simulink model "dyn"  (R2022a)
settings: Solver=VariableStepAuto  StartTime=0.0  StopTime=1.5  MaxStep=0.005  RelTol=1e-3
values from neighbouring files (symbols this model uses):
  A_1 = 0.0012    [WS.m]
  A_2 = 0.0012    [WS.m]
  D = [D_1 D_2 D_3 D_4 D_5 D_6]    [WS.m]
  E_1 = 8.25 * 10^4    (= 82500)    [WS.m]
  E_2 = 8.25 * 10^4    (= 82500)    [WS.m]
  g_x = 0.0    (= 0)    [WS.m]
  g_y = 0    [WS.m]
  g_z = 9.8    [WS.m]
  Gs_1 = E_1 / ( 2 * ( 1 + ni) )    (= 27684.5637584)    [WS.m]
  Gs_2 = E_2 / ( 2 *( 1 + ni) )    (= 27684.5637584)    [WS.m]
  Iax_1 = 1.0053e-07 * rate2    (= 9.55035e-08)    [WS.m]
  Iax_2 = 1.0053e-07 * rate2    (= 9.55035e-08)    [WS.m]
  Iay_1 = 1.0053e-07 * rate2    (= 9.55035e-08)    [WS.m]
  Iay_2 = 1.0053e-07 * rate2    (= 9.55035e-08)    [WS.m]
  Iaz_1 = 1.0053e-07 * rate2    (= 9.55035e-08)    [WS.m]
  Iaz_2 = 1.0053e-07 * rate2    (= 9.55035e-08)    [WS.m]
  Imx_1 = 10^-5 * rate1    (= 1e-05)    [WS.m]
  Imx_2 = 10^-5 * rate1    (= 1e-05)    [WS.m]
  Imy_1 = 10^-5 * rate1    (= 1e-05)    [WS.m]
  Imy_2 = 10^-5 * rate1    (= 1e-05)    [WS.m]
  Imz_1 = 10^-5 * rate1    (= 1e-05)    [WS.m]
  Imz_2 = 10^-5 * rate1    (= 1e-05)    [WS.m]
  l_1 = 0.05    [WS.m]
  l_2 = 0.05    [WS.m]
  m_1 = 0.08    [WS.m]
  m_2 = 0.08    [WS.m]
  p_tendon1_0 = [0.012,0,0]    [WS.m]
  p_tendon1_1 = [0.012,0,0]    [WS.m]
  p_tendon1_2 = [0.012,0,0]    [WS.m]
  p_tendon2_0 = [-0.012,0,0]    [WS.m]
  p_tendon2_1 = [-0.012,0,0]    [WS.m]
  p_tendon2_2 = [-0.012,0,0]    [WS.m]
  p_tendon3_0 = [0,0.012,0]    [WS.m]
  p_tendon3_1 = [0,0.012,0]    [WS.m]
  p_tendon3_2 = [0,0.012,0]    [WS.m]
  p_tendon4_0 = [0,-0.012,0]    [WS.m]
  p_tendon4_1 = [0,-0.012,0]    [WS.m]
  p_tendon4_2 = [0,-0.012,0]    [WS.m]
  p_tendon5_0 = [0.09,0,0]    [WS.m]
  p_tendon5_1 = [0.0636,0.0636,0]    [WS.m]
  p_tendon5_2 = [0,0.09,0]    [WS.m]
  x_0 = [0.001, 0.001 , 0.0 , 0 , 0.001,0]'    [WS.m]
  x_dot_0 = [0 , 0, 0, 0, 0, 0]'    [WS.m]
libraries: slpidlib x1, matrix_library x1
settings Model: Creator=atled  LastModifiedBy=atled

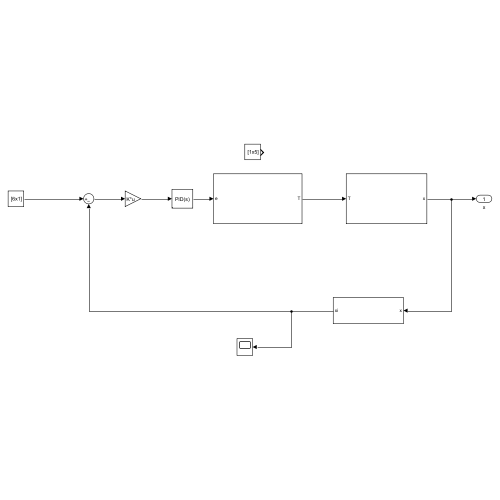
[thumbnail: Simulink's stored preview of the top-level diagram]
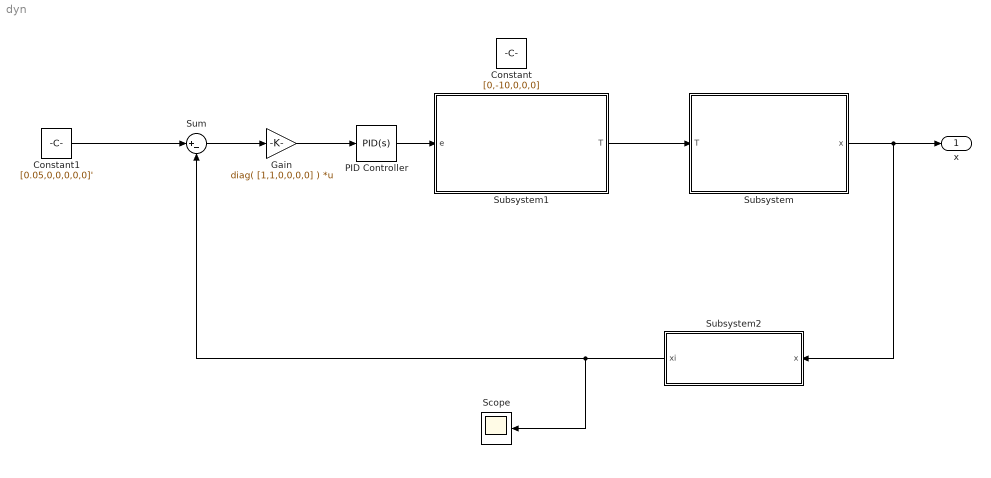
== system dyn ==
  Constant : Constant  Value=[0,-10,0,0,0]
  Constant1 : Constant  Value=[0.05,0,0,0,0,0]'  VectorParams1D=off
  Gain : Gain  Gain=diag( [1,1,0,0,0,0] )  Multiplication=Matrix(K*u)
  PID Controller : slpidlib/PID Controller  Controller=PID  Form=Parallel  TimeDomain=Continuous-time  UseExternalTs=off  SampleTime=-1  IntegratorMethod=Forward Euler  FilterMethod=Forward Euler  ControllerParametersSource=internal  P=0.2  I=0  UseKiTs=off  D=0  N=100  UseFilter=on  TunerSelectOption=Transfer Function Based (PID Tuner App)  InitialConditionSource=internal  InitialConditionForIntegrator=0  InitialConditionForFilter=0  DifferentiatorICPrevScaledInput=0  ExternalReset=none  TrackingMode=off  Kt=1  LimitOutput=off  SatLimitsSource=internal  UpperSaturationLimit=inf  LowerSaturationLimit=-inf  LinearizeAsGain=on  AntiWindupMode=none  Kb=1  POutMin=[]  POutMax=[]  IOutMin=[]  IOutMax=[]  DOutMin=[]  DOutMax=[]  NOutMin=[]  NOutMax=[]  SumOutMin=[]  SumOutMax=[]  SaturationOutMin=[]  SaturationOutMax=[]  PParamMin=[]  PParamMax=[]  IParamMin=[]  IParamMax=[]  DParamMin=[]  DParamMax=[]  NParamMin=[]  NParamMax=[]  KbParamMin=[]  KbParamMax=[]  KtParamMin=[]  KtParamMax=[]  KbOutMin=[]  KbOutMax=[]  KtOutMin=[]  KtOutMax=[]  IntegratorOutMin=[]  IntegratorOutMax=[]  FilterOutMin=[]  FilterOutMax=[]  SumI1OutMin=[]  SumI1OutMax=[]  SumI2OutMin=[]  SumI2OutMax=[]  SumI3OutMin=[]  SumI3OutMax=[]  SumI4OutMin=[]  SumI4OutMax=[]  SumDOutMin=[]  SumDOutMax=[]  DifferentiatorOutMin=[]  DifferentiatorOutMax=[]  FilterDiffOutCoefMin=[]  FilterDiffOutCoefMax=[]  ReciprocalOutMin=[]  ReciprocalOutMax=[]  SumDenOutMin=[]  SumDenOutMax=[]  SumNumOutMin=[]  SumNumOutMax=[]  DivideOutMin=[]  DivideOutMax=[]  UdiffTsProdOutMin=[]  UdiffTsProdOutMax=[]  NTsProdOutMin=[]  NTsProdOutMax=[]  UintegralTsProdOutMin=[]  UintegralTsProdOutMax=[]  UngainTsProdOutMin=[]  UngainTsProdOutMax=[]  IntegratorContinuousStateAttributes=''  IntegratorStateMustResolveToSignalObject=off  IntegratorRTWStateStorageClass=Auto  FilterContinuousStateAttributes=''  FilterStateMustResolveToSignalObject=off  FilterRTWStateStorageClass=Auto  ParallelPVariant=InternalParameters  IdealPVariant=Disabled  IVariant=InternalParameters  DVariant=InternalParameters  IntegratorVariant=Continuous  SatVariant=Disabled  AWVariant=Passthrough  PCopyVariant=Disabled  TRVariant=Disabled  FdbkBlocksVariant=Forward  IdealPFdbkVariant=Disabled  SatFdbkVariant=Disabled  DerivativeFilterVariant=ContFilter  NVariant=InternalParameters  NCopyVariant=Disabled  FilterICVariant=InternalICsFilter  IntegratorICVariant=InternalICs  ExternalResetVariant=Disabled  TRSumVariant=Passthrough  SumFdbkVariant=Disabled  SumVariant=Sum_PID  TsampFilterVariant=InternalTs  TsampNgainVariant=Passthrough  TsampIntegralVariant=Passthrough  ExternalSaturationOutDataTypeStr=Inherit: Same as second input  aMode=0
  Scope : Scope
  Subsystem : Subsystem
  Subsystem1 : Subsystem
  Subsystem2 : Subsystem
  Sum : Sum  Inputs=|+-
  x : Outport
  wires:
  Subsystem/1(x) -> Subsystem2/1(x), x/1
  Subsystem1/1(T) -> Subsystem/1(T)
  Constant1/1 -> Sum/1
  Subsystem2/1(xi) -> Sum/2, Scope/1
  Sum/1 -> Gain/1
  Gain/1 -> PID Controller/1
  PID Controller/1 -> Subsystem1/1(e)

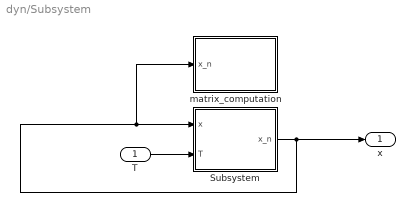
== system dyn/Subsystem ==
  T : Inport
  Subsystem : Subsystem
  matrix_computation : Subsystem
  x : Outport
  wires:
  Subsystem/1(x_n) -> x/1, matrix_computation/1(x_n), Subsystem/1(x)
  T/1 -> Subsystem/2(T)

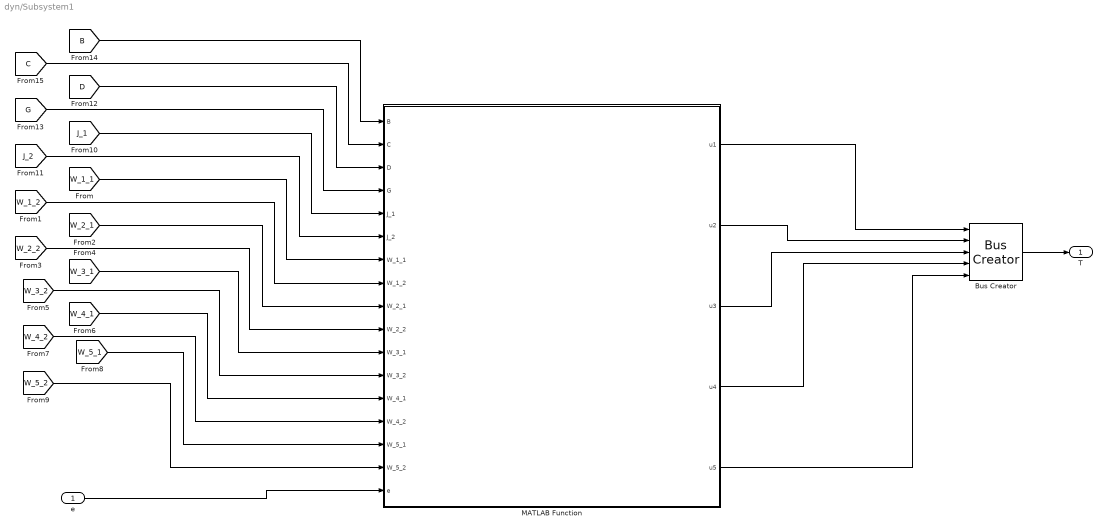
== system dyn/Subsystem1 ==
  e : Inport
  Bus Creator : BusCreator  Inputs=5
  MATLAB Function : MATLAB Function  TreatAsAtomicUnit=on
  T : Outport
  wires:
  [W_5_2] -> MATLAB Function/16(W_5_2)
  [W_4_1] -> MATLAB Function/13(W_4_1)
  [W_4_2] -> MATLAB Function/14(W_4_2)
  [J_2] -> MATLAB Function/6(J_2)
  [W_1_1] -> MATLAB Function/7(W_1_1)
  [G] -> MATLAB Function/4(G)
  [B] -> MATLAB Function/1(B)
  [J_1] -> MATLAB Function/5(J_1)
  [C] -> MATLAB Function/2(C)
  [D] -> MATLAB Function/3(D)
  [W_3_2] -> MATLAB Function/12(W_3_2)
  [W_2_2] -> MATLAB Function/10(W_2_2)
  e/1 -> MATLAB Function/17(e)
  [W_2_1] -> MATLAB Function/9(W_2_1)
  [W_3_1] -> MATLAB Function/11(W_3_1)
  [W_5_1] -> MATLAB Function/15(W_5_1)
  [W_1_2] -> MATLAB Function/8(W_1_2)
  MATLAB Function/1(u1) -> Bus Creator/1
  MATLAB Function/2(u2) -> Bus Creator/2
  MATLAB Function/3(u3) -> Bus Creator/3
  MATLAB Function/4(u4) -> Bus Creator/4
  MATLAB Function/5(u5) -> Bus Creator/5
  Bus Creator/1 -> T/1

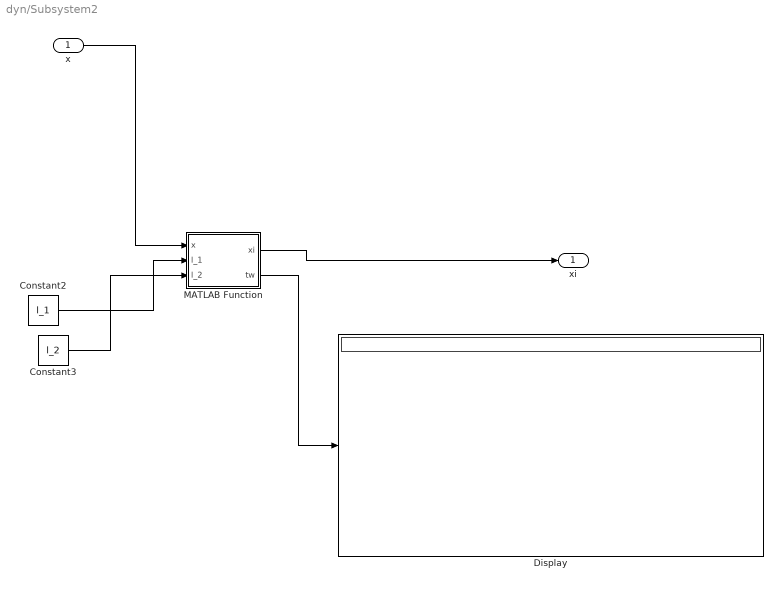
== system dyn/Subsystem2 ==
  x : Inport
  Constant2 : Constant  Value=l_1
  Constant3 : Constant  Value=l_2
  Display : Display
  MATLAB Function : MATLAB Function  TreatAsAtomicUnit=on
  xi : Outport
  wires:
  x/1 -> MATLAB Function/1(x)
  Constant3/1 -> MATLAB Function/3(l_2)
  MATLAB Function/1(xi) -> xi/1
  Constant2/1 -> MATLAB Function/2(l_1)
  MATLAB Function/2(tw) -> Display/1

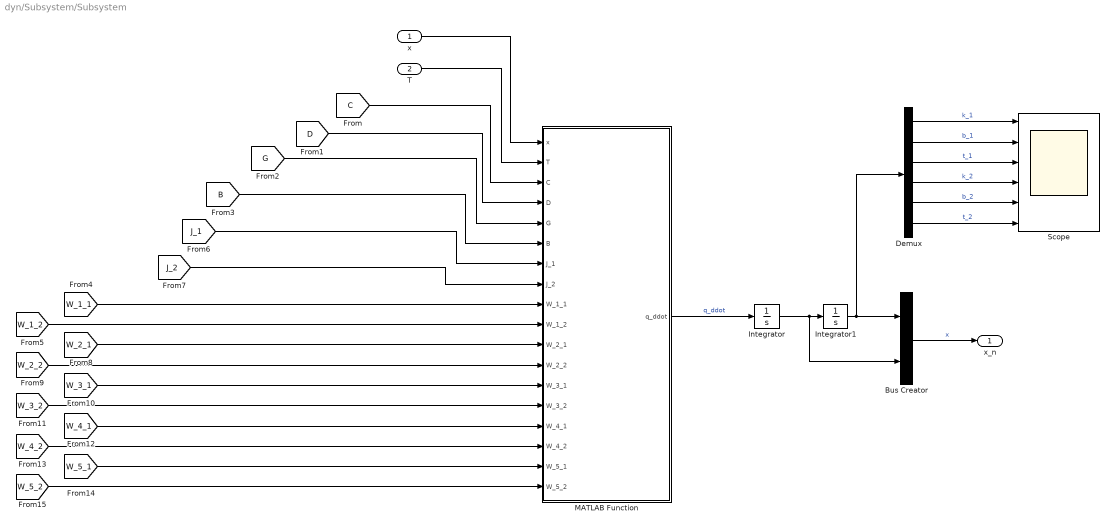
== system dyn/Subsystem/Subsystem ==
  x : Inport
  T : Inport  Port=2
  Bus Creator : BusCreator  Inputs=2
  Demux : Demux  Outputs=6
  Integrator : Integrator  InitialCondition=x_dot_0
  Integrator1 : Integrator  InitialCondition=x_0
  MATLAB Function : MATLAB Function  TreatAsAtomicUnit=on
  Scope : Scope  NumInputPorts=6
  x_n : Outport
  wires:
  T/1 -> MATLAB Function/2(T)
  x/1 -> MATLAB Function/1(x)
  Bus Creator/1 -> x_n/1  "x"
  [C] -> MATLAB Function/3(C)
  [D] -> MATLAB Function/4(D)
  [G] -> MATLAB Function/5(G)
  [B] -> MATLAB Function/6(B)
  MATLAB Function/1(q_ddot) -> Integrator/1  "q_ddot"
  Integrator/1 -> Integrator1/1, Bus Creator/2
  Integrator1/1 -> Demux/1, Bus Creator/1
  Demux/2 -> Scope/2  "b_1"
  Demux/1 -> Scope/1  "k_1"
  Demux/3 -> Scope/3  "t_1"
  Demux/4 -> Scope/4  "k_2"
  Demux/5 -> Scope/5  "b_2"
  Demux/6 -> Scope/6  "t_2"
  [W_1_1] -> MATLAB Function/9(W_1_1)
  [W_1_2] -> MATLAB Function/10(W_1_2)
  [J_1] -> MATLAB Function/7(J_1)
  [J_2] -> MATLAB Function/8(J_2)
  [W_2_1] -> MATLAB Function/11(W_2_1)
  [W_2_2] -> MATLAB Function/12(W_2_2)
  [W_3_1] -> MATLAB Function/13(W_3_1)
  [W_3_2] -> MATLAB Function/14(W_3_2)
  [W_4_1] -> MATLAB Function/15(W_4_1)
  [W_4_2] -> MATLAB Function/16(W_4_2)
  [W_5_1] -> MATLAB Function/17(W_5_1)
  [W_5_2] -> MATLAB Function/18(W_5_2)

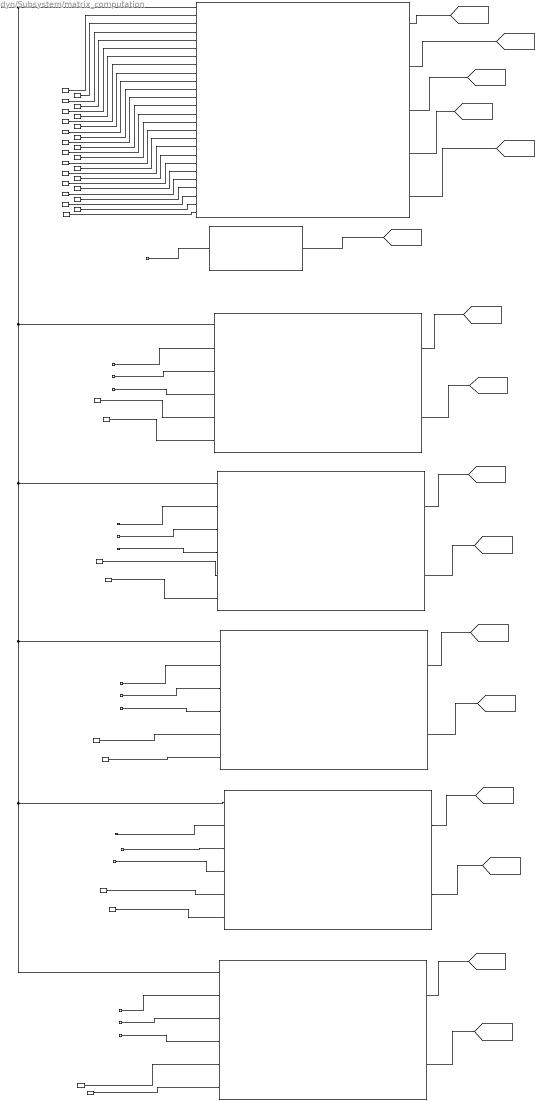
== system dyn/Subsystem/matrix_computation ==
  x_n : Inport
  Constant : Constant  Value=E_2
  Constant1 : Constant  Value=Gs_2
  Constant10 : Constant  Value=Imy_2
  Constant11 : Constant  Value=Imx_2
  Constant12 : Constant  Value=Imz_1
  Constant13 : Constant  Value=Imy_1
  Constant14 : Constant  Value=Imx_1
  Constant15 : Constant  Value=Iaz_1
  Constant16 : Constant  Value=Iay_1
  Constant17 : Constant  Value=Iax_1
  Constant18 : Constant  Value=Iaz_2
  Constant19 : Constant  Value=Iay_2
  Constant2 : Constant  Value=E_1
  Constant20 : Constant  Value=Iax_2
  Constant21 : Constant  Value=A_2
  Constant22 : Constant  Value=A_1
  Constant{23,26,31,33,35,37} (6 alike) : Constant  Value=l_2
  Constant{24,27,32,34,36,38} (6 alike) : Constant  Value=l_1
  Constant25 : Constant  Value=D
  Constant28 : Constant  Value=p_tendon1_0
  Constant29 : Constant  Value=p_tendon1_1
  Constant3 : Constant  Value=Gs_1
  Constant30 : Constant  Value=p_tendon1_2
  Constant39 : Constant  Value=p_tendon2_0
  Constant4 : Constant  Value=g_z
  Constant40 : Constant  Value=p_tendon2_1
  Constant41 : Constant  Value=p_tendon2_2
  Constant42 : Constant  Value=p_tendon3_0
  Constant43 : Constant  Value=p_tendon3_1
  Constant44 : Constant  Value=p_tendon3_2
  Constant45 : Constant  Value=p_tendon4_0
  Constant46 : Constant  Value=p_tendon4_1
  Constant47 : Constant  Value=p_tendon4_2
  Constant48 : Constant  Value=p_tendon5_0
  Constant49 : Constant  Value=p_tendon5_1
  Constant5 : Constant  Value=g_y
  Constant50 : Constant  Value=p_tendon5_2
  Constant6 : Constant  Value=g_x
  Constant7 : Constant  Value=m_2
  Constant8 : Constant  Value=m_1
  Constant9 : Constant  Value=Imz_2
  Create Diagonal Matrix : matrix_library/Create Diagonal Matrix
      settings: SourceProductBaseCode=SL
  MATLAB Function : MATLAB Function  TreatAsAtomicUnit=on
  MATLAB Function1 : MATLAB Function  TreatAsAtomicUnit=on
  MATLAB Function2 : MATLAB Function  TreatAsAtomicUnit=on
  MATLAB Function3 : MATLAB Function  TreatAsAtomicUnit=on
  MATLAB Function4 : MATLAB Function  TreatAsAtomicUnit=on
  MATLAB Function5 : MATLAB Function  TreatAsAtomicUnit=on
  tag scope: B=global, C=global, D=global, G=global, J_1=global, J_2=global, W_1_1=global, W_1_2=global, W_2_1=global, W_2_2=global, W_3_1=global, W_3_2=global, W_4_1=global, W_4_2=global, W_5_1=global, W_5_2=global
  wires:
  Constant17/1 -> MATLAB Function/9(Iax_1)
  Constant3/1 -> MATLAB Function/23(Gs_1)
  Constant19/1 -> MATLAB Function/7(Iay_2)
  MATLAB Function/3(G_m) -> [G]
  Constant22/1 -> MATLAB Function/4(A_1)
  Constant9/1 -> MATLAB Function/17(Imz_2)
  Constant8/1 -> MATLAB Function/18(m_1)
  Constant24/1 -> MATLAB Function/2(l_1)
  Constant2/1 -> MATLAB Function/24(E_1)
  Constant4/1 -> MATLAB Function/22(g_z)
  MATLAB Function/5(J_1_m) -> [J_1]
  Constant16/1 -> MATLAB Function/10(Iay_1)
  Constant20/1 -> MATLAB Function/6(Iax_2)
  MATLAB Function/2(B_m) -> [B]
  Constant6/1 -> MATLAB Function/20(g_x)
  Constant15/1 -> MATLAB Function/11(Iaz_1)
  Constant14/1 -> MATLAB Function/12(Imx_1)
  Constant1/1 -> MATLAB Function/25(Gs_2)
  Constant23/1 -> MATLAB Function/3(l_2)
  Constant10/1 -> MATLAB Function/16(Imy_2)
  MATLAB Function/4(J_2_m) -> [J_2]
  Constant12/1 -> MATLAB Function/14(Imz_1)
  MATLAB Function/1(C_m) -> [C]
  Constant5/1 -> MATLAB Function/21(g_y)
  Constant11/1 -> MATLAB Function/15(Imx_2)
  Constant7/1 -> MATLAB Function/19(m_2)
  Constant18/1 -> MATLAB Function/8(Iaz_2)
  Constant13/1 -> MATLAB Function/13(Imy_1)
  Constant21/1 -> MATLAB Function/5(A_2)
  Constant/1 -> MATLAB Function/26(E_2)
  Create Diagonal Matrix/1 -> [D]
  Constant25/1 -> Create Diagonal Matrix/1
  x_n/1 -> MATLAB Function/1(x), MATLAB Function5/1(x), MATLAB Function4/1(x), MATLAB Function2/1(x), MATLAB Function1/1(x), MATLAB Function3/1(x)
  Constant27/1 -> MATLAB Function3/5(l_1)
  Constant26/1 -> MATLAB Function3/6(l_2)
  Constant28/1 -> MATLAB Function3/2(p_tendon_0)
  Constant29/1 -> MATLAB Function3/3(p_tendon_1)
  Constant30/1 -> MATLAB Function3/4(p_tendon_2)
  MATLAB Function3/1(W1) -> [W_1_1]
  MATLAB Function3/2(W2) -> [W_1_2]
  Constant31/1 -> MATLAB Function1/6(l_2)
  Constant32/1 -> MATLAB Function1/5(l_1)
  Constant33/1 -> MATLAB Function2/6(l_2)
  Constant34/1 -> MATLAB Function2/5(l_1)
  Constant35/1 -> MATLAB Function5/6(l_2)
  Constant36/1 -> MATLAB Function5/5(l_1)
  Constant37/1 -> MATLAB Function4/6(l_2)
  Constant38/1 -> MATLAB Function4/5(l_1)
  MATLAB Function1/2(W2) -> [W_2_2]
  MATLAB Function1/1(W1) -> [W_2_1]
  MATLAB Function2/2(W2) -> [W_3_2]
  MATLAB Function2/1(W1) -> [W_3_1]
  MATLAB Function4/2(W2) -> [W_4_2]
  MATLAB Function4/1(W1) -> [W_4_1]
  MATLAB Function5/2(W2) -> [W_5_2]
  MATLAB Function5/1(W1) -> [W_5_1]
  Constant39/1 -> MATLAB Function1/2(p_tendon_0)
  Constant40/1 -> MATLAB Function1/3(p_tendon_1)
  Constant41/1 -> MATLAB Function1/4(p_tendon_2)
  Constant44/1 -> MATLAB Function2/4(p_tendon_2)
  Constant43/1 -> MATLAB Function2/3(p_tendon_1)
  Constant42/1 -> MATLAB Function2/2(p_tendon_0)
  Constant47/1 -> MATLAB Function4/4(p_tendon_2)
  Constant46/1 -> MATLAB Function4/3(p_tendon_1)
  Constant45/1 -> MATLAB Function4/2(p_tendon_0)
  Constant50/1 -> MATLAB Function5/4(p_tendon_2)
  Constant49/1 -> MATLAB Function5/3(p_tendon_1)
  Constant48/1 -> MATLAB Function5/2(p_tendon_0)

== matlab function dyn/Subsystem/matrix_computation/MATLAB Function1 ==
  data: x input; W1 output; p_tendon_0 input; p_tendon_1 input; p_tendon_2 input; l_1 input; l_2 input; W2 output
function [W1,W2] = fcn(x,p_tendon_0,p_tendon_1,p_tendon_2,l_1,l_2)
k_1= x(1);
b_1=x(2);
t_1=x(3);
k_2=x(4);
b_2=x(5);
t_2=x(6);
k_dot_1=x(7);
b_dot_1=x(8);
t_dot_1=x(9);
k_dot_2=x(10);
b_dot_2=x(11);
t_dot_2=x(12);

T_0 = eye(4);
T_1m = t_epcc_sym_corr([l_1,0,k_1/l_1,b_1/l_1,t_1/l_1]');
T_2m = T_1m * t_epcc_sym_corr([l_2,0,k_2/l_2,b_2/l_2,t_2/l_2]');

O_0 = T_0(1:3,4);
O_1 = T_1m(1:3,4);
O_2 = T_2m(1:3,4);

P_1_0 = O_0 + p_tendon_0;
P_1_1 = O_1 + p_tendon_1;
P_1_2 = O_2 + p_tendon_2;

O0O1 = vectord(O_0,O_1);
O1O2 = vectord(O_1,O_2);

O0P0 = vectord(O_0,P_1_0);
O1P1 = vectord(O_1,P_1_1);
O2P2 = vectord(O_2,P_1_2);

P0P1 = vectord(P_1_0,P_1_1);
P1P2 = vectord(P_1_1,P_1_2);

W1 = zeros(6,1);
W2 = zeros(6,1);

F2 = P1P2 / norm(P1P2);

W2(1:3,1) = F2  ;
W2(4:6,1) = cross_form(O2P2) * F2 + cross_form( O1O2 ) * F2 ;


F2 = P1P2 / norm(P1P2);

W2(1:3,1) = F2  ;
W2(4:6,1) = cross_form(O2P2) * F2 + cross_form( O1O2 ) * F2 ;


F1 = - P0P1 / norm(P0P1) + P1P2 / norm(P1P2);
W1(1:3,1) = F1 + F2;
W1(4:6,1) = cross_form(O1P1) * (F1) + cross_form( O0O1 ) * F1 + W2(4:6,1);

== matlab function dyn/Subsystem/matrix_computation/MATLAB Function2 ==
  data: x input; W1 output; p_tendon_0 input; p_tendon_1 input; p_tendon_2 input; l_1 input; l_2 input; W2 output
function [W1,W2] = fcn(x,p_tendon_0,p_tendon_1,p_tendon_2,l_1,l_2)
k_1= x(1);
b_1=x(2);
t_1=x(3);
k_2=x(4);
b_2=x(5);
t_2=x(6);
k_dot_1=x(7);
b_dot_1=x(8);
t_dot_1=x(9);
k_dot_2=x(10);
b_dot_2=x(11);
t_dot_2=x(12);

T_0 = eye(4);
T_1m = t_epcc_sym_corr([l_1,0,k_1/l_1,b_1/l_1,t_1/l_1]');
T_2m = T_1m * t_epcc_sym_corr([l_2,0,k_2/l_2,b_2/l_2,t_2/l_2]');

O_0 = T_0(1:3,4);
O_1 = T_1m(1:3,4);
O_2 = T_2m(1:3,4);

P_1_0 = O_0 + p_tendon_0;
P_1_1 = O_1 + p_tendon_1;
P_1_2 = O_2 + p_tendon_2;

O0O1 = vectord(O_0,O_1);
O1O2 = vectord(O_1,O_2);

O0P0 = vectord(O_0,P_1_0);
O1P1 = vectord(O_1,P_1_1);
O2P2 = vectord(O_2,P_1_2);

P0P1 = vectord(P_1_0,P_1_1);
P1P2 = vectord(P_1_1,P_1_2);

W1 = zeros(6,1);
W2 = zeros(6,1);

F2 = P1P2 / norm(P1P2);

W2(1:3,1) = F2  ;
W2(4:6,1) = cross_form(O2P2) * F2 + cross_form( O1O2 ) * F2 ;


F2 = P1P2 / norm(P1P2);

W2(1:3,1) = F2  ;
W2(4:6,1) = cross_form(O2P2) * F2 + cross_form( O1O2 ) * F2 ;


F1 = - P0P1 / norm(P0P1) + P1P2 / norm(P1P2);
W1(1:3,1) = F1 + F2;
W1(4:6,1) = cross_form(O1P1) * (F1) + cross_form( O0O1 ) * F1 + W2(4:6,1);

== matlab function dyn/Subsystem/matrix_computation/MATLAB Function3 ==
  data: x input; W1 output; p_tendon_0 input; p_tendon_1 input; p_tendon_2 input; l_1 input; l_2 input; W2 output
function [W1,W2] = fcn(x,p_tendon_0,p_tendon_1,p_tendon_2,l_1,l_2)
k_1= x(1);
b_1=x(2);
t_1=x(3);
k_2=x(4);
b_2=x(5);
t_2=x(6);
k_dot_1=x(7);
b_dot_1=x(8);
t_dot_1=x(9);
k_dot_2=x(10);
b_dot_2=x(11);
t_dot_2=x(12);

T_0 = eye(4);
T_1m = t_epcc_sym_corr([l_1,0,k_1/l_1,b_1/l_1,t_1/l_1]');
T_2m = T_1m * t_epcc_sym_corr([l_2,0,k_2/l_2,b_2/l_2,t_2/l_2]');

O_0 = T_0(1:3,4);
O_1 = T_1m(1:3,4);
O_2 = T_2m(1:3,4);

P_1_0 = O_0 + p_tendon_0;
P_1_1 = O_1 + p_tendon_1;
P_1_2 = O_2 + p_tendon_2;

O0O1 = vectord(O_0,O_1);
O1O2 = vectord(O_1,O_2);

O0P0 = vectord(O_0,P_1_0);
O1P1 = vectord(O_1,P_1_1);
O2P2 = vectord(O_2,P_1_2);

P0P1 = vectord(P_1_0,P_1_1);
P1P2 = vectord(P_1_1,P_1_2);

W1 = zeros(6,1);
W2 = zeros(6,1);

F2 = P1P2 / norm(P1P2);

W2(1:3,1) = F2  ;
W2(4:6,1) = cross_form(O2P2) * F2 + cross_form( O1O2 ) * F2 ;


F2 = P1P2 / norm(P1P2);

W2(1:3,1) = F2  ;
W2(4:6,1) = cross_form(O2P2) * F2 + cross_form( O1O2 ) * F2 ;


F1 = - P0P1 / norm(P0P1) + P1P2 / norm(P1P2);
W1(1:3,1) = F1 + F2;
W1(4:6,1) = cross_form(O1P1) * (F1) + cross_form( O0O1 ) * F1 + W2(4:6,1);

== matlab function dyn/Subsystem/matrix_computation/MATLAB Function4 ==
  data: x input; W1 output; p_tendon_0 input; p_tendon_1 input; p_tendon_2 input; l_1 input; l_2 input; W2 output
function [W1,W2] = fcn( x,p_tendon_0,p_tendon_1,p_tendon_2,l_1,l_2)
k_1= x(1);
b_1=x(2);
t_1=x(3);
k_2=x(4);
b_2=x(5);
t_2=x(6);
k_dot_1=x(7);
b_dot_1=x(8);
t_dot_1=x(9);
k_dot_2=x(10);
b_dot_2=x(11);
t_dot_2=x(12);

T_0 = eye(4);
T_1m = t_epcc_sym_corr([l_1,0,k_1/l_1,b_1/l_1,t_1/l_1]');
T_2m = T_1m * t_epcc_sym_corr([l_2,0,k_2/l_2,b_2/l_2,t_2/l_2]');

O_0 = T_0(1:3,4);
O_1 = T_1m(1:3,4);
O_2 = T_2m(1:3,4);

P_1_0 = O_0 + p_tendon_0;
P_1_1 = O_1 + p_tendon_1;
P_1_2 = O_2 + p_tendon_2;

O0O1 = vectord(O_0,O_1);
O1O2 = vectord(O_1,O_2);

O0P0 = vectord(O_0,P_1_0);
O1P1 = vectord(O_1,P_1_1);
O2P2 = vectord(O_2,P_1_2);

P0P1 = vectord(P_1_0,P_1_1);
P1P2 = vectord(P_1_1,P_1_2);

W1 = zeros(6,1);
W2 = zeros(6,1);

F2 = P1P2 / norm(P1P2);

W2(1:3,1) = F2  ;
W2(4:6,1) = cross_form(O2P2) * F2 + cross_form( O1O2 ) * F2 ;


F2 = P1P2 / norm(P1P2);

W2(1:3,1) = F2  ;
W2(4:6,1) = cross_form(O2P2) * F2 + cross_form( O1O2 ) * F2 ;


F1 = - P0P1 / norm(P0P1) + P1P2 / norm(P1P2);
W1(1:3,1) = F1 + F2;
W1(4:6,1) = cross_form(O1P1) * (F1) + cross_form( O0O1 ) * F1 + W2(4:6,1);

== matlab function dyn/Subsystem/matrix_computation/MATLAB Function5 ==
  data: x input; W1 output; p_tendon_0 input; p_tendon_1 input; p_tendon_2 input; l_1 input; l_2 input; W2 output
function [W1,W2] = fcn(x,p_tendon_0,p_tendon_1,p_tendon_2,l_1,l_2)
k_1= x(1);
b_1=x(2);
t_1=x(3);
k_2=x(4);
b_2=x(5);
t_2=x(6);
k_dot_1=x(7);
b_dot_1=x(8);
t_dot_1=x(9);
k_dot_2=x(10);
b_dot_2=x(11);
t_dot_2=x(12);

T_0 = eye(4);
T_1m = t_epcc_sym_corr([l_1,0,k_1/l_1,b_1/l_1,t_1/l_1]');
T_2m = T_1m * t_epcc_sym_corr([l_2,0,k_2/l_2,b_2/l_2,t_2/l_2]');

O_0 = T_0(1:3,4);
O_1 = T_1m(1:3,4);
O_2 = T_2m(1:3,4);

P_1_0 = O_0 + p_tendon_0;
P_1_1 = O_1 + p_tendon_1;
P_1_2 = O_2 + p_tendon_2;


O0P0 = vectord(O_0,P_1_0);
O1P1 = vectord(O_1,P_1_1);
O2P2 = vectord(O_2,P_1_2);

O0O1 = vectord(O_0,O_1);
O1O2 = vectord(O_1,O_2);

P0P1 = vectord(P_1_0,P_1_1);
P1P2 = vectord(P_1_1,P_1_2);

W1 = zeros(6,1);
W2 = zeros(6,1);

F2 = P1P2 / norm(P1P2);

W2(1:3,1) = F2  ;
W2(4:6,1) = cross_form(O2P2) * F2 + cross_form( O1O2 ) * F2 ;


F2 = P1P2 / norm(P1P2);

W2(1:3,1) = F2  ;
W2(4:6,1) = cross_form(O2P2) * F2 + cross_form( O1O2 ) * F2 ;


F1 = - P0P1 / norm(P0P1) + P1P2 / norm(P1P2);
W1(1:3,1) = F1 + F2;
W1(4:6,1) = cross_form(O1P1) * (F1) + cross_form( O0O1 ) * F1 + W2(4:6,1);

== matlab function dyn/Subsystem1/MATLAB Function ==
  data: B input; u1 output; C input; D input; G input; J_1 input; J_2 input; W_1_1 input; W_1_2 input; W_2_1 input; W_2_2 input; W_3_1 input; W_3_2 input; W_4_1 input; W_4_2 input; W_5_1 input; W_5_2 input; u2 output; e input; u3 output; u4 output; u5 output
function [u1,u2,u3,u4,u5] = fcn(B,C,D,G,J_1,J_2,W_1_1,W_1_2, W_2_1,W_2_2, W_3_1,W_3_2, W_4_1,W_4_2, W_5_1,W_5_2,e)
A1 = [ J_1(1:6,:)' * W_1_1(1:6,1) , J_2(1:6,:)' * W_1_2(1:6,1) ];
% A2 = [ J_1(1:6,1)' * W_2_1(1:6,2) ; J_2(1:6,2)' * W_2_2(1:6,2) ];
% A3 = [ J_1(1:6,1)' * W_3_1(1:6,2) ; J_2(1:6,2)' * W_3_2(1:6,2) ];
% A4 = [ J_1(1:6,1)' * W_4_1(1:6,2) ; J_2(1:6,2)' * W_4_2(1:6,2) ];
% A5 = [ J_1(1:6,1)' * W_5_1(1:6,2) ; J_2(1:6,2)' * W_5_2(1:6,2) ];


J = [ J_2(1,:) ; J_2(2,:) ; J_2(6,:) ];
A1
J_2*e
u1 = pinv(A1) * ( J_2 * e );
u2 = 0;%ppinv(A2) * ( J_2 * e );
u3 = 0;%ppinv(A3) * ( J_2 * e );
u4 = 0;%ppinv(A4) * ( J_2 * e );
u5 = 0;%ppinv(A5) * ( J_2 * e );

== matlab function dyn/Subsystem2/MATLAB Function ==
  data: x input; xi output; l_1 input; l_2 input; tw output
function [xi,tw] = fcn(x,l_1,l_2)
k_1= x(1);
b_1=x(2);
t_1=x(3);
k_2=x(4);
b_2=x(5);
t_2=x(6);
k_dot_1=x(7);
b_dot_1=x(8);
t_dot_1=x(9);
k_dot_2=x(10);
b_dot_2=x(11);
t_dot_2=x(12);

t1 = t_epcc_sym_corr([l_1,0,k_1/l_1^2,b_1/l_1^2,t_1]');
t2 = t_epcc_sym_corr([l_2,0,k_2/l_2^2,b_2/l_2^2,t_2]');
tw = (t1*t2);
vx = tw(1,4) ;
vy = tw(2,4) ;
vz = tw(3,4) ;
ux = tw(3,2) ;
uy = tw(1,3) ;
uz = tw(2,1) ;

xi = [vx ; vy ; vz ; ux ; uy ; uz ] ;
tw

== matlab function dyn/Subsystem/Subsystem/MATLAB Function ==
  data: x input; T input; q_ddot output; C input; D input; G input; B input; J_1 input; J_2 input; W_1_1 input; W_1_2 input; W_2_1 input; W_2_2 input; W_3_1 input; W_3_2 input; W_4_1 input; W_4_2 input; W_5_1 input; W_5_2 input
function q_ddot  = fcn(x,T,C,D,G,B,J_1,J_2,W_1_1,W_1_2,W_2_1,W_2_2,W_3_1,W_3_2,W_4_1,W_4_2,W_5_1,W_5_2)
q = x(1:6);
q_dot = x(7:12);
T1 = T(1);
T2 =T(2);
T3 =T(3);
T4 =T(4);
T5 =T(5);
A1 = [ J_1(1:6,1:3)' * W_1_1 ; J_2(1:6,4:6)' * W_1_2 ];
A2 = [ J_1(1:6,1:3)' * W_2_1 ; J_2(1:6,4:6)' * W_2_2 ];
A3 = [ J_1(1:6,1:3)' * W_3_1 ; J_2(1:6,4:6)' * W_3_2 ];
A4 = [ J_1(1:6,1:3)' * W_4_1 ; J_2(1:6,4:6)' * W_4_2 ];
A5 = [ J_1(1:6,1:3)' * W_5_1 ; J_2(1:6,4:6)' * W_5_2 ];
q_ddot = - B^-1 * (C * q_dot + D* q_dot + G  - A1 * (-T1) - A2 * (-T2) - A3 * (-T3) - A4 * (-T4) - A5 * (-T5)) ;

== matlab function dyn/Subsystem/matrix_computation/MATLAB Function ==
  data: C_m output; x input; l_1 input; l_2 input; A_1 input; A_2 input; Iax_2 input; Iay_2 input; Iaz_2 input; Iax_1 input; Iay_1 input; Iaz_1 input; Imx_1 input; Imy_1 input; Imz_1 input; Imx_2 input; Imy_2 input; Imz_2 input; m_1 input; m_2 input; g_x input; g_y input; g_z input; Gs_1 input; E_1 input; Gs_2 input; E_2 input; B_m output; G_m output; J_2_m output; J_1_m output
function [C_m, B_m, G_m , J_2_m, J_1_m]  = fcn(x,l_1,l_2,A_1,A_2,Iax_2,Iay_2,Iaz_2,Iax_1,Iay_1,Iaz_1,Imx_1,Imy_1,Imz_1,Imx_2,Imy_2,Imz_2,m_1,m_2,g_x,g_y,g_z,Gs_1,E_1,Gs_2,E_2)
k_1= x(1);
b_1=x(2);
t_1=x(3);
k_2=x(4);
b_2=x(5);
t_2=x(6);
k_dot_1=x(7);
b_dot_1=x(8);
t_dot_1=x(9);
k_dot_2=x(10);
b_dot_2=x(11);
t_dot_2=x(12);


B_m = B(k_1,b_1,t_1,k_2,b_2,t_2,k_dot_1,b_dot_1,t_dot_1,k_dot_2,b_dot_2,t_dot_2,l_1,l_2,A_1,A_2,Iax_2,Iay_2,Iaz_2,Iax_1,Iay_1,Iaz_1,Imx_1,Imy_1,Imz_1,Imx_2,Imy_2,Imz_2,m_1,m_2,g_x,g_y,g_z,Gs_1,E_1,Gs_2,E_2);
G_m = G(k_1,b_1,t_1,k_2,b_2,t_2,k_dot_1,b_dot_1,t_dot_1,k_dot_2,b_dot_2,t_dot_2,l_1,l_2,A_1,A_2,Iax_2,Iay_2,Iaz_2,Iax_1,Iay_1,Iaz_1,Imx_1,Imy_1,Imz_1,Imx_2,Imy_2,Imz_2,m_1,m_2,g_x,g_y,g_z,Gs_1,E_1,Gs_2,E_2);
J_2_m = J_2(b_1,b_2,k_1,k_2,l_1,l_2,t_1,t_2);
J_1_m = J_1(b_1,k_1,l_1,t_1);


C11m = C11(k_1,b_1,t_1,k_2,b_2,t_2,k_dot_1,b_dot_1,t_dot_1,k_dot_2,b_dot_2,t_dot_2,l_1,l_2,A_1,A_2,Iax_2,Iay_2,Iaz_2,Iax_1,Iay_1,Iaz_1,Imx_1,Imy_1,Imz_1,Imx_2,Imy_2,Imz_2,m_1,m_2,g_x,g_y,g_z,Gs_1,E_1,Gs_2,E_2);
C12m = C12(k_1,b_1,t_1,k_2,b_2,t_2,k_dot_1,b_dot_1,t_dot_1,k_dot_2,b_dot_2,t_dot_2,l_1,l_2,A_1,A_2,Iax_2,Iay_2,Iaz_2,Iax_1,Iay_1,Iaz_1,Imx_1,Imy_1,Imz_1,Imx_2,Imy_2,Imz_2,m_1,m_2,g_x,g_y,g_z,Gs_1,E_1,Gs_2,E_2);
C13m = C13(k_1,b_1,t_1,k_2,b_2,t_2,k_dot_1,b_dot_1,t_dot_1,k_dot_2,b_dot_2,t_dot_2,l_1,l_2,A_1,A_2,Iax_2,Iay_2,Iaz_2,Iax_1,Iay_1,Iaz_1,Imx_1,Imy_1,Imz_1,Imx_2,Imy_2,Imz_2,m_1,m_2,g_x,g_y,g_z,Gs_1,E_1,Gs_2,E_2);
C14m = C14(k_1,b_1,t_1,k_2,b_2,t_2,k_dot_1,b_dot_1,t_dot_1,k_dot_2,b_dot_2,t_dot_2,l_1,l_2,A_1,A_2,Iax_2,Iay_2,Iaz_2,Iax_1,Iay_1,Iaz_1,Imx_1,Imy_1,Imz_1,Imx_2,Imy_2,Imz_2,m_1,m_2,g_x,g_y,g_z,Gs_1,E_1,Gs_2,E_2);
C15m = C15(k_1,b_1,t_1,k_2,b_2,t_2,k_dot_1,b_dot_1,t_dot_1,k_dot_2,b_dot_2,t_dot_2,l_1,l_2,A_1,A_2,Iax_2,Iay_2,Iaz_2,Iax_1,Iay_1,Iaz_1,Imx_1,Imy_1,Imz_1,Imx_2,Imy_2,Imz_2,m_1,m_2,g_x,g_y,g_z,Gs_1,E_1,Gs_2,E_2);
C16m = C16(k_1,b_1,t_1,k_2,b_2,t_2,k_dot_1,b_dot_1,t_dot_1,k_dot_2,b_dot_2,t_dot_2,l_1,l_2,A_1,A_2,Iax_2,Iay_2,Iaz_2,Iax_1,Iay_1,Iaz_1,Imx_1,Imy_1,Imz_1,Imx_2,Imy_2,Imz_2,m_1,m_2,g_x,g_y,g_z,Gs_1,E_1,Gs_2,E_2);

C21m = C21(k_1,b_1,t_1,k_2,b_2,t_2,k_dot_1,b_dot_1,t_dot_1,k_dot_2,b_dot_2,t_dot_2,l_1,l_2,A_1,A_2,Iax_2,Iay_2,Iaz_2,Iax_1,Iay_1,Iaz_1,Imx_1,Imy_1,Imz_1,Imx_2,Imy_2,Imz_2,m_1,m_2,g_x,g_y,g_z,Gs_1,E_1,Gs_2,E_2);
C22m = C22(k_1,b_1,t_1,k_2,b_2,t_2,k_dot_1,b_dot_1,t_dot_1,k_dot_2,b_dot_2,t_dot_2,l_1,l_2,A_1,A_2,Iax_2,Iay_2,Iaz_2,Iax_1,Iay_1,Iaz_1,Imx_1,Imy_1,Imz_1,Imx_2,Imy_2,Imz_2,m_1,m_2,g_x,g_y,g_z,Gs_1,E_1,Gs_2,E_2);
C23m = C23(k_1,b_1,t_1,k_2,b_2,t_2,k_dot_1,b_dot_1,t_dot_1,k_dot_2,b_dot_2,t_dot_2,l_1,l_2,A_1,A_2,Iax_2,Iay_2,Iaz_2,Iax_1,Iay_1,Iaz_1,Imx_1,Imy_1,Imz_1,Imx_2,Imy_2,Imz_2,m_1,m_2,g_x,g_y,g_z,Gs_1,E_1,Gs_2,E_2);
C24m = C24(k_1,b_1,t_1,k_2,b_2,t_2,k_dot_1,b_dot_1,t_dot_1,k_dot_2,b_dot_2,t_dot_2,l_1,l_2,A_1,A_2,Iax_2,Iay_2,Iaz_2,Iax_1,Iay_1,Iaz_1,Imx_1,Imy_1,Imz_1,Imx_2,Imy_2,Imz_2,m_1,m_2,g_x,g_y,g_z,Gs_1,E_1,Gs_2,E_2);
C25m = C25(k_1,b_1,t_1,k_2,b_2,t_2,k_dot_1,b_dot_1,t_dot_1,k_dot_2,b_dot_2,t_dot_2,l_1,l_2,A_1,A_2,Iax_2,Iay_2,Iaz_2,Iax_1,Iay_1,Iaz_1,Imx_1,Imy_1,Imz_1,Imx_2,Imy_2,Imz_2,m_1,m_2,g_x,g_y,g_z,Gs_1,E_1,Gs_2,E_2);
C26m = C26(k_1,b_1,t_1,k_2,b_2,t_2,k_dot_1,b_dot_1,t_dot_1,k_dot_2,b_dot_2,t_dot_2,l_1,l_2,A_1,A_2,Iax_2,Iay_2,Iaz_2,Iax_1,Iay_1,Iaz_1,Imx_1,Imy_1,Imz_1,Imx_2,Imy_2,Imz_2,m_1,m_2,g_x,g_y,g_z,Gs_1,E_1,Gs_2,E_2);

C31m = C31(k_1,b_1,t_1,k_2,b_2,t_2,k_dot_1,b_dot_1,t_dot_1,k_dot_2,b_dot_2,t_dot_2,l_1,l_2,A_1,A_2,Iax_2,Iay_2,Iaz_2,Iax_1,Iay_1,Iaz_1,Imx_1,Imy_1,Imz_1,Imx_2,Imy_2,Imz_2,m_1,m_2,g_x,g_y,g_z,Gs_1,E_1,Gs_2,E_2);
C32m = C32(k_1,b_1,t_1,k_2,b_2,t_2,k_dot_1,b_dot_1,t_dot_1,k_dot_2,b_dot_2,t_dot_2,l_1,l_2,A_1,A_2,Iax_2,Iay_2,Iaz_2,Iax_1,Iay_1,Iaz_1,Imx_1,Imy_1,Imz_1,Imx_2,Imy_2,Imz_2,m_1,m_2,g_x,g_y,g_z,Gs_1,E_1,Gs_2,E_2);
C33m = C33(k_1,b_1,t_1,k_2,b_2,t_2,k_dot_1,b_dot_1,t_dot_1,k_dot_2,b_dot_2,t_dot_2,l_1,l_2,A_1,A_2,Iax_2,Iay_2,Iaz_2,Iax_1,Iay_1,Iaz_1,Imx_1,Imy_1,Imz_1,Imx_2,Imy_2,Imz_2,m_1,m_2,g_x,g_y,g_z,Gs_1,E_1,Gs_2,E_2);
C34m = C34(k_1,b_1,t_1,k_2,b_2,t_2,k_dot_1,b_dot_1,t_dot_1,k_dot_2,b_dot_2,t_dot_2,l_1,l_2,A_1,A_2,Iax_2,Iay_2,Iaz_2,Iax_1,Iay_1,Iaz_1,Imx_1,Imy_1,Imz_1,Imx_2,Imy_2,Imz_2,m_1,m_2,g_x,g_y,g_z,Gs_1,E_1,Gs_2,E_2);
C35m = C35(k_1,b_1,t_1,k_2,b_2,t_2,k_dot_1,b_dot_1,t_dot_1,k_dot_2,b_dot_2,t_dot_2,l_1,l_2,A_1,A_2,Iax_2,Iay_2,Iaz_2,Iax_1,Iay_1,Iaz_1,Imx_1,Imy_1,Imz_1,Imx_2,Imy_2,Imz_2,m_1,m_2,g_x,g_y,g_z,Gs_1,E_1,Gs_2,E_2);
C36m = C36(k_1,b_1,t_1,k_2,b_2,t_2,k_dot_1,b_dot_1,t_dot_1,k_dot_2,b_dot_2,t_dot_2,l_1,l_2,A_1,A_2,Iax_2,Iay_2,Iaz_2,Iax_1,Iay_1,Iaz_1,Imx_1,Imy_1,Imz_1,Imx_2,Imy_2,Imz_2,m_1,m_2,g_x,g_y,g_z,Gs_1,E_1,Gs_2,E_2);

C41m = C41(k_1,b_1,t_1,k_2,b_2,t_2,k_dot_1,b_dot_1,t_dot_1,k_dot_2,b_dot_2,t_dot_2,l_1,l_2,A_1,A_2,Iax_2,Iay_2,Iaz_2,Iax_1,Iay_1,Iaz_1,Imx_1,Imy_1,Imz_1,Imx_2,Imy_2,Imz_2,m_1,m_2,g_x,g_y,g_z,Gs_1,E_1,Gs_2,E_2);
C42m = C42(k_1,b_1,t_1,k_2,b_2,t_2,k_dot_1,b_dot_1,t_dot_1,k_dot_2,b_dot_2,t_dot_2,l_1,l_2,A_1,A_2,Iax_2,Iay_2,Iaz_2,Iax_1,Iay_1,Iaz_1,Imx_1,Imy_1,Imz_1,Imx_2,Imy_2,Imz_2,m_1,m_2,g_x,g_y,g_z,Gs_1,E_1,Gs_2,E_2);
C43m = C43(k_1,b_1,t_1,k_2,b_2,t_2,k_dot_1,b_dot_1,t_dot_1,k_dot_2,b_dot_2,t_dot_2,l_1,l_2,A_1,A_2,Iax_2,Iay_2,Iaz_2,Iax_1,Iay_1,Iaz_1,Imx_1,Imy_1,Imz_1,Imx_2,Imy_2,Imz_2,m_1,m_2,g_x,g_y,g_z,Gs_1,E_1,Gs_2,E_2);
C44m = C44(k_1,b_1,t_1,k_2,b_2,t_2,k_dot_1,b_dot_1,t_dot_1,k_dot_2,b_dot_2,t_dot_2,l_1,l_2,A_1,A_2,Iax_2,Iay_2,Iaz_2,Iax_1,Iay_1,Iaz_1,Imx_1,Imy_1,Imz_1,Imx_2,Imy_2,Imz_2,m_1,m_2,g_x,g_y,g_z,Gs_1,E_1,Gs_2,E_2);
C45m = C45(k_1,b_1,t_1,k_2,b_2,t_2,k_dot_1,b_dot_1,t_dot_1,k_dot_2,b_dot_2,t_dot_2,l_1,l_2,A_1,A_2,Iax_2,Iay_2,Iaz_2,Iax_1,Iay_1,Iaz_1,Imx_1,Imy_1,Imz_1,Imx_2,Imy_2,Imz_2,m_1,m_2,g_x,g_y,g_z,Gs_1,E_1,Gs_2,E_2);
C46m = C46(k_1,b_1,t_1,k_2,b_2,t_2,k_dot_1,b_dot_1,t_dot_1,k_dot_2,b_dot_2,t_dot_2,l_1,l_2,A_1,A_2,Iax_2,Iay_2,Iaz_2,Iax_1,Iay_1,Iaz_1,Imx_1,Imy_1,Imz_1,Imx_2,Imy_2,Imz_2,m_1,m_2,g_x,g_y,g_z,Gs_1,E_1,Gs_2,E_2);

C51m = C51(k_1,b_1,t_1,k_2,b_2,t_2,k_dot_1,b_dot_1,t_dot_1,k_dot_2,b_dot_2,t_dot_2,l_1,l_2,A_1,A_2,Iax_2,Iay_2,Iaz_2,Iax_1,Iay_1,Iaz_1,Imx_1,Imy_1,Imz_1,Imx_2,Imy_2,Imz_2,m_1,m_2,g_x,g_y,g_z,Gs_1,E_1,Gs_2,E_2);
C52m = C52(k_1,b_1,t_1,k_2,b_2,t_2,k_dot_1,b_dot_1,t_dot_1,k_dot_2,b_dot_2,t_dot_2,l_1,l_2,A_1,A_2,Iax_2,Iay_2,Iaz_2,Iax_1,Iay_1,Iaz_1,Imx_1,Imy_1,Imz_1,Imx_2,Imy_2,Imz_2,m_1,m_2,g_x,g_y,g_z,Gs_1,E_1,Gs_2,E_2);
C53m = C53(k_1,b_1,t_1,k_2,b_2,t_2,k_dot_1,b_dot_1,t_dot_1,k_dot_2,b_dot_2,t_dot_2,l_1,l_2,A_1,A_2,Iax_2,Iay_2,Iaz_2,Iax_1,Iay_1,Iaz_1,Imx_1,Imy_1,Imz_1,Imx_2,Imy_2,Imz_2,m_1,m_2,g_x,g_y,g_z,Gs_1,E_1,Gs_2,E_2);
C54m = C54(k_1,b_1,t_1,k_2,b_2,t_2,k_dot_1,b_dot_1,t_dot_1,k_dot_2,b_dot_2,t_dot_2,l_1,l_2,A_1,A_2,Iax_2,Iay_2,Iaz_2,Iax_1,Iay_1,Iaz_1,Imx_1,Imy_1,Imz_1,Imx_2,Imy_2,Imz_2,m_1,m_2,g_x,g_y,g_z,Gs_1,E_1,Gs_2,E_2);
C55m = C55(k_1,b_1,t_1,k_2,b_2,t_2,k_dot_1,b_dot_1,t_dot_1,k_dot_2,b_dot_2,t_dot_2,l_1,l_2,A_1,A_2,Iax_2,Iay_2,Iaz_2,Iax_1,Iay_1,Iaz_1,Imx_1,Imy_1,Imz_1,Imx_2,Imy_2,Imz_2,m_1,m_2,g_x,g_y,g_z,Gs_1,E_1,Gs_2,E_2);
C56m = C56(k_1,b_1,t_1,k_2,b_2,t_2,k_dot_1,b_dot_1,t_dot_1,k_dot_2,b_dot_2,t_dot_2,l_1,l_2,A_1,A_2,Iax_2,Iay_2,Iaz_2,Iax_1,Iay_1,Iaz_1,Imx_1,Imy_1,Imz_1,Imx_2,Imy_2,Imz_2,m_1,m_2,g_x,g_y,g_z,Gs_1,E_1,Gs_2,E_2);

C61m = C61(k_1,b_1,t_1,k_2,b_2,t_2,k_dot_1,b_dot_1,t_dot_1,k_dot_2,b_dot_2,t_dot_2,l_1,l_2,A_1,A_2,Iax_2,Iay_2,Iaz_2,Iax_1,Iay_1,Iaz_1,Imx_1,Imy_1,Imz_1,Imx_2,Imy_2,Imz_2,m_1,m_2,g_x,g_y,g_z,Gs_1,E_1,Gs_2,E_2);
C62m = C62(k_1,b_1,t_1,k_2,b_2,t_2,k_dot_1,b_dot_1,t_dot_1,k_dot_2,b_dot_2,t_dot_2,l_1,l_2,A_1,A_2,Iax_2,Iay_2,Iaz_2,Iax_1,Iay_1,Iaz_1,Imx_1,Imy_1,Imz_1,Imx_2,Imy_2,Imz_2,m_1,m_2,g_x,g_y,g_z,Gs_1,E_1,Gs_2,E_2);
C63m = C63(k_1,b_1,t_1,k_2,b_2,t_2,k_dot_1,b_dot_1,t_dot_1,k_dot_2,b_dot_2,t_dot_2,l_1,l_2,A_1,A_2,Iax_2,Iay_2,Iaz_2,Iax_1,Iay_1,Iaz_1,Imx_1,Imy_1,Imz_1,Imx_2,Imy_2,Imz_2,m_1,m_2,g_x,g_y,g_z,Gs_1,E_1,Gs_2,E_2);
C64m = C64(k_1,b_1,t_1,k_2,b_2,t_2,k_dot_1,b_dot_1,t_dot_1,k_dot_2,b_dot_2,t_dot_2,l_1,l_2,A_1,A_2,Iax_2,Iay_2,Iaz_2,Iax_1,Iay_1,Iaz_1,Imx_1,Imy_1,Imz_1,Imx_2,Imy_2,Imz_2,m_1,m_2,g_x,g_y,g_z,Gs_1,E_1,Gs_2,E_2);
C65m = C65(k_1,b_1,t_1,k_2,b_2,t_2,k_dot_1,b_dot_1,t_dot_1,k_dot_2,b_dot_2,t_dot_2,l_1,l_2,A_1,A_2,Iax_2,Iay_2,Iaz_2,Iax_1,Iay_1,Iaz_1,Imx_1,Imy_1,Imz_1,Imx_2,Imy_2,Imz_2,m_1,m_2,g_x,g_y,g_z,Gs_1,E_1,Gs_2,E_2);
C66m = C66(k_1,b_1,t_1,k_2,b_2,t_2,k_dot_1,b_dot_1,t_dot_1,k_dot_2,b_dot_2,t_dot_2,l_1,l_2,A_1,A_2,Iax_2,Iay_2,Iaz_2,Iax_1,Iay_1,Iaz_1,Imx_1,Imy_1,Imz_1,Imx_2,Imy_2,Imz_2,m_1,m_2,g_x,g_y,g_z,Gs_1,E_1,Gs_2,E_2);


C_m = [C11m C12m C13m C14m C15m C16m ; 
    C21m C22m C23m C24m C25m C26m;
    C31m C32m C33m C34m C35m C36m;
    C41m C42m C43m C44m C45m C46m;
    C51m C52m C53m C54m C55m C56m;
    C61m C62m C63m C64m C65m C66m];
